simulink model "process_plant_model_4dof"  (R2020a)
settings: Solver=VariableStepAuto  StartTime=0.0  StopTime=10.0  RelTol=1e-3
values from neighbouring files (symbols this model uses):
  B_aug = [b11 b12 b13 b14 b15 b16 ... (first row only)    [constants.m]
  B_psinv_aug = B_aug'/(B_aug*B_aug')    [constants.m]
  coriolis_effect = 1    [run_simulation.m]    (also in run_simulation_STA_controller.m; run_simulation_dp_model.m)
  d_11 = 250    [constants.m]    (also in constants_dp_model.m; constants_model_coriolis.m; constants_process_model.m)
  d_22 = 200    [constants.m]    (also in constants_dp_model.m; constants_model_coriolis.m; constants_process_model.m)
  d_33 = 175    [constants.m]    (also in constants_dp_model.m; constants_model_coriolis.m; constants_process_model.m)
  d_66 = 15    [constants.m]    (also in constants_process_model.m)
  d_n11 = 350    [constants.m]
  d_n22 = 350    [constants.m]
  d_n33 = 400    [constants.m]
  d_n66 = 75    [constants.m]
  g_z = 9.81    [run_simulation_FL_controller.m]    (also in run_simulation_PID_controller.m = 0.91; run_simulation_SM_controller.m = 0.91; run_simulation_STA_controller.m = 0.91; run_simulation_dp_model.m = 0.91)
  m_11 = m_RB11+m_A11    (= 144)    [constants.m]    (also in constants_dp_model.m; constants_model_coriolis.m; constants_process_model.m)
  m_22 = m_RB22+m_A22    (= 162)    [constants.m]    (also in constants_dp_model.m; constants_model_coriolis.m; constants_process_model.m)
  m_A11 = 54    [constants.m]    (also in constants_dp_model.m; constants_model_coriolis.m; constants_process_model.m)
  m_A22 = 72    [constants.m]    (also in constants_dp_model.m; constants_model_coriolis.m; constants_process_model.m)
  m_A33 = 360    [constants.m]    (also in constants_dp_model.m; constants_model_coriolis.m; constants_process_model.m)
  m_A66 = 5.2    [constants.m]    (also in constants_process_model.m)
  m_RB11 = 90    [constants.m]    (also in constants_dp_model.m; constants_model_coriolis.m; constants_process_model.m)
  m_RB22 = 90    [constants.m]    (also in constants_dp_model.m; constants_model_coriolis.m; constants_process_model.m)
  m_RB33 = 90    [constants.m]    (also in constants_dp_model.m; constants_model_coriolis.m; constants_process_model.m)
  m_RB66 = 13    [constants.m]    (also in constants_process_model.m)
  nonlinear_damping = 1    [run_simulation.m]    (also in run_simulation_STA_controller.m; run_simulation_dp_model.m)
  psi0 = deg2rad(psi0)    [constants.m]    (also in constants_dp_model.m; constants_model_coriolis.m; constants_process_model.m)
  r0 = 0    [constants.m]    (also in constants_dp_model.m; constants_model_coriolis.m; constants_process_model.m)
  u0 = 0    [constants.m]    (also in constants_dp_model.m; constants_model_coriolis.m; constants_process_model.m)
  v0 = 0    [constants.m]    (also in constants_dp_model.m; constants_model_coriolis.m; constants_process_model.m)
  w0 = 0    [constants.m]    (also in constants_dp_model.m; constants_model_coriolis.m; constants_process_model.m)
  x0 = -2*50    (= -100)    [constants.m]    (also in constants_dp_model.m = 0; constants_model_coriolis.m = 0; constants_process_model.m = 0)
  y0 = 0    [constants.m]    (also in constants_dp_model.m; constants_model_coriolis.m; constants_process_model.m)
  z0 = 0    [constants.m]    (also in constants_dp_model.m; constants_model_coriolis.m; constants_process_model.m)
settings Model: Creator=kenng  LastModifiedBy=kennyhn

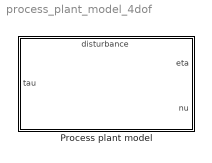
== system process_plant_model_4dof ==
  Process plant model : Subsystem
      settings: PortSchema="{\"entries\":[{\"content\":{\"sides\":[{\"content\":{\"connectorIds\":[\"In1\"]},\"type\":\"ConnectorPlacement.EquallySpacedRectSide\",\"uuid\":\"e717a587-3200-458e-ba24-dd41565550b9\"},{\"content\":{\"connectorIds\":[\"Out1\",\"Out2\"],\"side\":\"RIGHT\"},\"type\":\"ConnectorPlacement.EquallySpacedRectSide\",\"uuid\":\"302c9cc9-c34e-45c2-bf93-40982187bd66\"},{\"content\":{\"connectorIds\":[\"In2\"],\"side\":\"TOP\"},\"type\":\"ConnectorPlacement.EquallySpacedRectSide\",\"uuid\":\"4b1c13ad-6fa1-447d-8a08-ad292496a8ea\"}]},\"type\":\"ConnectorPlacement.EquallySpacedConnector\",\"uuid\":\"78ff5622-69b9-4402-ac71-5e2cc2861626\"}],\"packageUris\":[\"http://schema.mathworks.com/mf0/Connector/19700101\"],\"version\":\"1.0\"}"

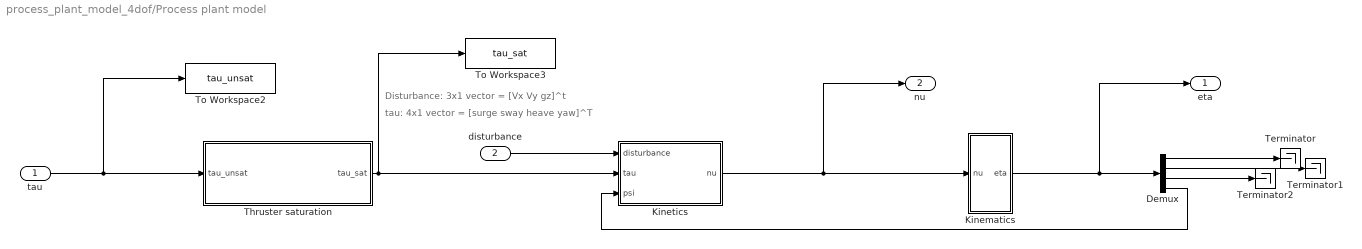
== system process_plant_model_4dof/Process plant model ==
  note: tau: 4x1 vector = [surge sway heave yaw]^T
  note: Disturbance: 3x1 vector = [Vx Vy gz]^t
  tau : Inport
  disturbance : Inport  Port=2
  Demux : Demux
  Kinematics : Subsystem
  Kinetics : Subsystem
  Terminator : Terminator
  Terminator1 : Terminator
  Terminator2 : Terminator
  Thruster saturation : Subsystem
  To Workspace2 : ToWorkspace  VariableName=tau_unsat  SaveFormat=Structure With Time  SampleTime=-1
  To Workspace3 : ToWorkspace  VariableName=tau_sat  SaveFormat=Structure With Time  SampleTime=-1
  eta : Outport
  nu : Outport  Port=2
  wires:
  Kinetics/1(nu) -> nu/1, Kinematics/1(nu)
  Demux/4 -> Kinetics/3(psi)
  Demux/2 -> Terminator1/1
  Kinematics/1(eta) -> eta/1, Demux/1
  Demux/1 -> Terminator/1
  Demux/3 -> Terminator2/1
  disturbance/1 -> Kinetics/1(disturbance)
  Thruster saturation/1(tau_sat) -> Kinetics/2(tau), To Workspace3/1
  tau/1 -> Thruster saturation/1(tau_unsat), To Workspace2/1

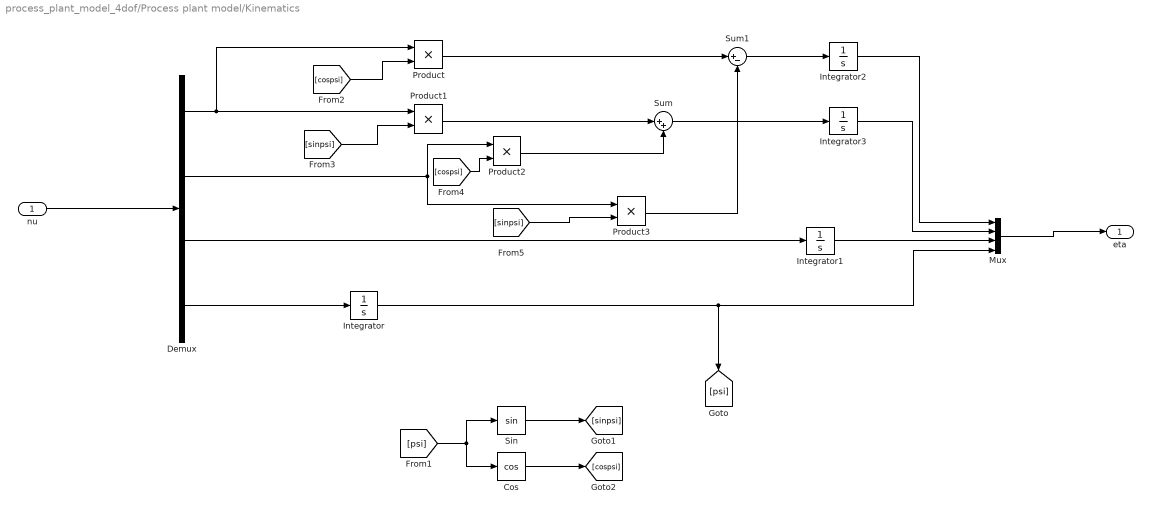
== system process_plant_model_4dof/Process plant model/Kinematics ==
  nu : Inport
  Cos : Trigonometry  Operator=cos
  Demux : Demux
  Integrator : Integrator  InitialCondition=psi0
  Integrator1 : Integrator  InitialCondition=z0
  Integrator2 : Integrator  InitialCondition=x0
  Integrator3 : Integrator  InitialCondition=y0
  Mux : Mux
  Product{,1..3} (4 alike) : Product
  Sin : Trigonometry
  Sum : Sum  Inputs=|++
  Sum1 : Sum  Inputs=|+-
  eta : Outport
  wires:
  Sin/1 -> [sinpsi]
  Demux/3 -> Integrator1/1
  Demux/1 -> Product1/1, Product/1
  Demux/2 -> Product3/1, Product2/1
  [sinpsi] -> Product3/2
  [psi] -> Sin/1, Cos/1
  [cospsi] -> Product2/2
  Cos/1 -> [cospsi]
  Product1/1 -> Sum/1
  Integrator/1 -> Mux/4, [psi]
  [sinpsi] -> Product1/2
  Product/1 -> Sum1/1
  Sum1/1 -> Integrator2/1
  Demux/4 -> Integrator/1
  Sum/1 -> Integrator3/1
  [cospsi] -> Product/2
  nu/1 -> Demux/1
  Product2/1 -> Sum/2
  Product3/1 -> Sum1/2
  Integrator3/1 -> Mux/2
  Integrator1/1 -> Mux/3
  Integrator2/1 -> Mux/1
  Mux/1 -> eta/1

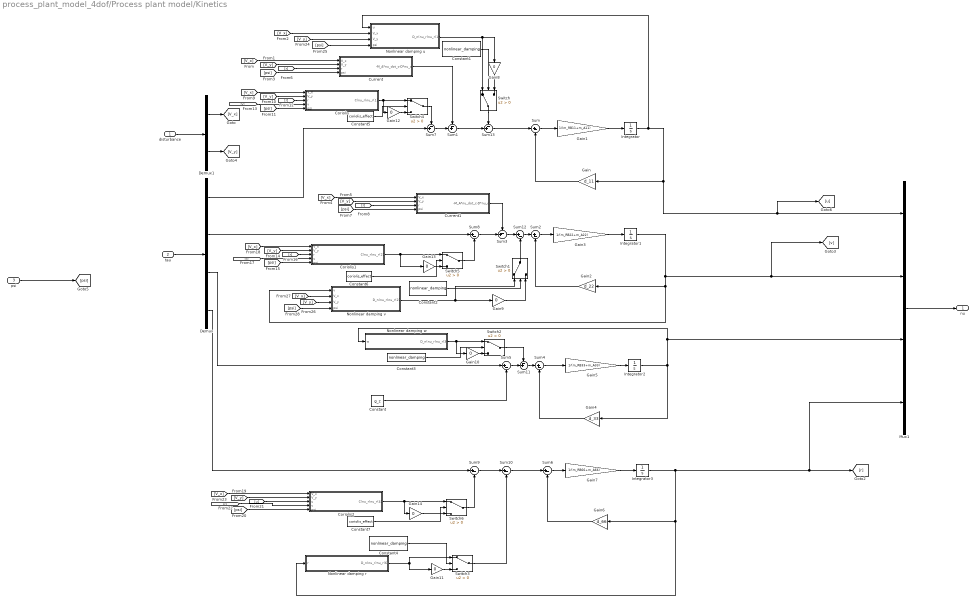
== system process_plant_model_4dof/Process plant model/Kinetics ==
  disturbance : Inport
  tau : Inport  Port=2
  psi : Inport  Port=3
  Constant : Constant  Value=g_z
  Constant{1..4} (4 alike) : Constant  Value=nonlinear_damping
  Constant5 : Constant  Value=coriolis_effect
  Constant6 : Constant  Value=coriolis_effect
  Constant7 : Constant  Value=coriolis_effect
  Coriolis : Subsystem
  Coriolis1 : Subsystem
  Coriolis2 : Subsystem
  Current : Subsystem
  Current1 : Subsystem
  Demux : Demux
  Demux1 : Demux  Outputs=2
  Gain : Gain  Gain=d_11
  Gain1 : Gain  Gain=1/(m_RB11+m_A11)
  Gain{8..14} (7 alike) : Gain  Gain=0
  Gain2 : Gain  Gain=d_22
  Gain3 : Gain  Gain=1/(m_RB22+m_A22)
  Gain4 : Gain  Gain=d_33
  Gain5 : Gain  Gain=1/(m_RB33+m_A33)
  Gain6 : Gain  Gain=d_66
  Gain7 : Gain  Gain=1/(m_RB66+m_A66)
  Integrator : Integrator  InitialCondition=u0
  Integrator1 : Integrator  InitialCondition=v0
  Integrator2 : Integrator  InitialCondition=w0
  Integrator3 : Integrator  InitialCondition=r0
  Mux1 : Mux
  Nonlinear damping r : Subsystem
  Nonlinear damping u : Subsystem
  Nonlinear damping v : Subsystem
  Nonlinear damping w : Subsystem
  Sum{,2,4..6,8..10,12} (9 alike) : Sum  Inputs=|+-
  Sum{1,3,7,11,13} (5 alike) : Sum  Inputs=-+|
  Switch{,1..6} (7 alike) : Switch  Criteria=u2 > Threshold
  nu : Outport
  wires:
  Demux1/1 -> [V_x]
  Gain1/1 -> Integrator/1
  Sum/1 -> Gain1/1
  tau/1 -> Demux/1
  Integrator1/1 -> Nonlinear damping v/1(v), Gain2/1, [v], Mux1/2
  Gain3/1 -> Integrator1/1
  Mux1/1 -> nu/1
  Integrator/1 -> Nonlinear damping u/1(u), [u], Mux1/1, Gain/1
  Integrator2/1 -> Gain4/1, Nonlinear damping w/1(w), Mux1/3
  Gain5/1 -> Integrator2/1
  Sum4/1 -> Gain5/1
  Gain2/1 -> Sum2/2
  Sum2/1 -> Gain3/1
  Gain/1 -> Sum/2
  Gain4/1 -> Sum4/2
  Gain6/1 -> Sum6/2
  Demux1/2 -> [V_y]
  [r] -> Current/3(r)
  Integrator3/1 -> [r], Mux1/4, Nonlinear damping r/1(r), Gain6/1
  disturbance/1 -> Demux1/1
  Sum6/1 -> Gain7/1
  Gain7/1 -> Integrator3/1
  psi/1 -> [psi]
  Current/1(-M_A*nu_dot_c-D*nu_c) -> Sum1/1
  [V_y] -> Current/2(V_y)
  [V_x] -> Current/1(V_x)
  [psi] -> Current/4(psi)
  [r] -> Current1/3(r)
  [psi] -> Current1/4(psi)
  [V_x] -> Current1/1(V_x)
  [V_y] -> Current1/2(V_y)
  Current1/1(-M_A*nu_dot_c-D*nu_c) -> Sum3/1
  Constant/1 -> Sum5/2
  Demux/3 -> Sum5/1
  Demux/1 -> Sum7/2
  Sum7/1 -> Sum1/2
  [V_x] -> Coriolis/1(V_x)
  [psi] -> Coriolis/5(psi)
  [r] -> Coriolis/3(r)
  [V_y] -> Coriolis/2(V_y)
  [v] -> Coriolis/4(v)
  [u] -> Coriolis1/4(u)
  [V_y] -> Coriolis1/2(V_y)
  [psi] -> Coriolis1/5(psi)
  [V_x] -> Coriolis1/1(V_x)
  [r] -> Coriolis1/3(r)
  Sum8/1 -> Sum3/2
  Demux/2 -> Sum8/1
  [v] -> Coriolis2/4(v)
  [V_y] -> Coriolis2/2(V_y)
  [psi] -> Coriolis2/5(psi)
  [V_x] -> Coriolis2/1(V_x)
  [u] -> Coriolis2/3(u)
  Demux/4 -> Sum9/1
  Sum10/1 -> Sum6/1
  Sum5/1 -> Sum11/2
  Sum11/1 -> Sum4/1
  Nonlinear damping w/1(D_n(nu_r)nu_r(3)) -> Gain10/1, Switch2/1
  Sum12/1 -> Sum2/1
  Sum1/1 -> Sum13/2
  Sum13/1 -> Sum/1
  Nonlinear damping u/1(D_n(nu_r)nu_r(1)) -> Switch/1, Gain8/1
  [V_x] -> Nonlinear damping u/2(V_x)
  [V_y] -> Nonlinear damping u/3(V_y)
  [psi] -> Nonlinear damping u/4(psi)
  Sum3/1 -> Sum12/1
  Nonlinear damping v/1(D_n(nu_r)nu_r(2)) -> Gain9/1, Switch1/1
  [V_x] -> Nonlinear damping v/2(V_x)
  [V_y] -> Nonlinear damping v/3(V_y)
  [psi] -> Nonlinear damping v/4(psi)
  Sum9/1 -> Sum10/1
  Switch/1 -> Sum13/1
  Switch1/1 -> Sum12/2
  Switch2/1 -> Sum11/1
  Switch3/1 -> Sum10/2
  Constant1/1 -> Switch/2
  Gain8/1 -> Switch/3
  Gain9/1 -> Switch1/3
  Constant2/1 -> Switch1/2
  Gain10/1 -> Switch2/3
  Constant3/1 -> Switch2/2
  Gain11/1 -> Switch3/3
  Constant4/1 -> Switch3/2
  Nonlinear damping r/1(D_n(nu_r)nu_r(6)) -> Switch3/1, Gain11/1
  Switch4/1 -> Sum7/1
  Coriolis/1(C(nu_r)nu_r(1)) -> Switch4/1, Gain12/1
  Constant5/1 -> Switch4/2
  Gain12/1 -> Switch4/3
  Switch5/1 -> Sum8/2
  Gain13/1 -> Switch5/3
  Constant6/1 -> Switch5/2
  Coriolis1/1(C(nu_r)nu_r(2)) -> Switch5/1, Gain13/1
  Coriolis2/1(C(nu_r)nu_r(4)) -> Switch6/1, Gain14/1
  Switch6/1 -> Sum9/2
  Gain14/1 -> Switch6/3
  Constant7/1 -> Switch6/2

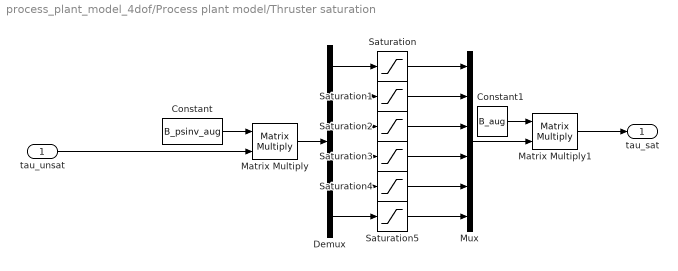
== system process_plant_model_4dof/Process plant model/Thruster saturation ==
  tau_unsat : Inport
  Constant : Constant  Value=B_psinv_aug
  Constant1 : Constant  Value=B_aug
  Demux : Demux  Outputs=6
  Matrix Multiply : Product  Multiplication=Matrix(*)
  Matrix Multiply1 : Product  Multiplication=Matrix(*)
  Mux : Mux  Inputs=6
  Saturation{,1..5} (6 alike) : Saturate  UpperLimit=120  LowerLimit=-120
  tau_sat : Outport
  wires:
  tau_unsat/1 -> Matrix Multiply/2
  Constant/1 -> Matrix Multiply/1
  Matrix Multiply/1 -> Demux/1
  Demux/2 -> Saturation1/1
  Demux/1 -> Saturation/1
  Demux/3 -> Saturation2/1
  Demux/4 -> Saturation3/1
  Demux/5 -> Saturation4/1
  Demux/6 -> Saturation5/1
  Saturation/1 -> Mux/1
  Saturation1/1 -> Mux/2
  Saturation2/1 -> Mux/3
  Saturation3/1 -> Mux/4
  Saturation4/1 -> Mux/5
  Saturation5/1 -> Mux/6
  Mux/1 -> Matrix Multiply1/2
  Constant1/1 -> Matrix Multiply1/1
  Matrix Multiply1/1 -> tau_sat/1

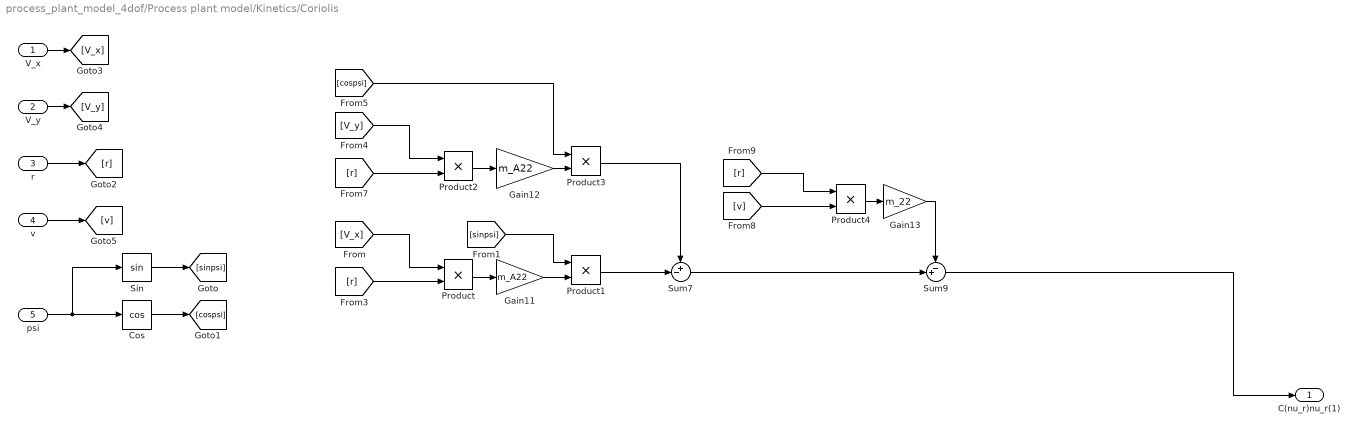
== system process_plant_model_4dof/Process plant model/Kinetics/Coriolis ==
  V_x : Inport
  V_y : Inport  Port=2
  r : Inport  Port=3
  v : Inport  Port=4
  psi : Inport  Port=5
  Cos : Trigonometry  Operator=cos
  Gain11 : Gain  Gain=m_A22
  Gain12 : Gain  Gain=m_A22
  Gain13 : Gain  Gain=m_22
  Product{,1..4} (5 alike) : Product
  Sin : Trigonometry
  Sum7 : Sum  Inputs=+-|
  Sum9 : Sum  Inputs=-+|
  C(nu_r)nu_r(1) : Outport
  wires:
  Gain11/1 -> Product1/2
  Product2/1 -> Gain12/1
  [cospsi] -> Product3/1
  [r] -> Product2/2
  [v] -> Product4/2
  Product4/1 -> Gain13/1
  [V_x] -> Product/1
  Product3/1 -> Sum7/1
  Gain12/1 -> Product3/2
  Product/1 -> Gain11/1
  [V_y] -> Product2/1
  [r] -> Product/2
  Product1/1 -> Sum7/2
  [sinpsi] -> Product1/1
  Sum7/1 -> Sum9/2
  [r] -> Product4/1
  Sum9/1 -> C(nu_r)nu_r(1)/1
  psi/1 -> Sin/1, Cos/1
  Sin/1 -> [sinpsi]
  Cos/1 -> [cospsi]
  r/1 -> [r]
  V_x/1 -> [V_x]
  V_y/1 -> [V_y]
  v/1 -> [v]
  Gain13/1 -> Sum9/1

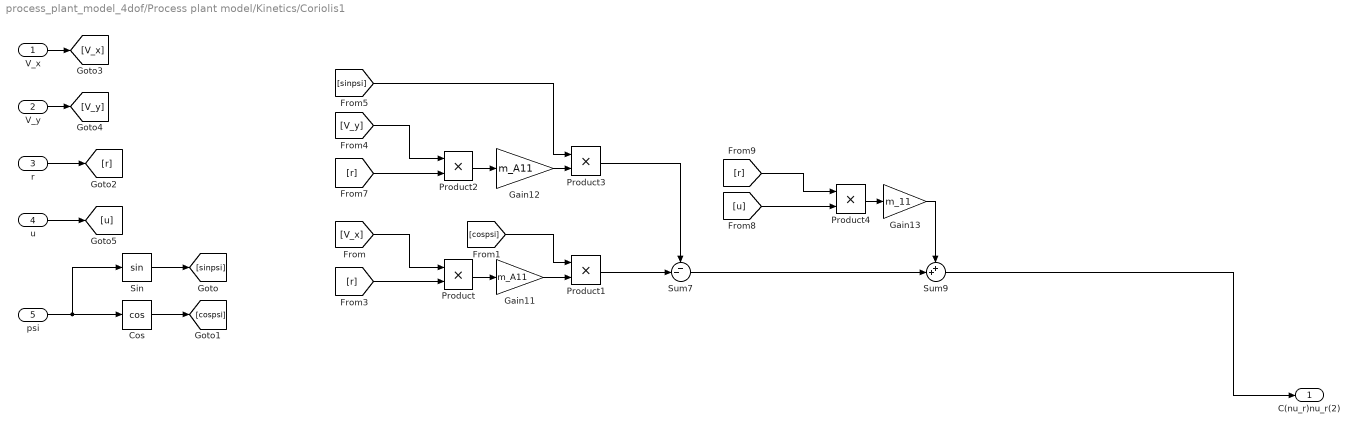
== system process_plant_model_4dof/Process plant model/Kinetics/Coriolis1 ==
  V_x : Inport
  V_y : Inport  Port=2
  r : Inport  Port=3
  u : Inport  Port=4
  psi : Inport  Port=5
  Cos : Trigonometry  Operator=cos
  Gain11 : Gain  Gain=m_A11
  Gain12 : Gain  Gain=m_A11
  Gain13 : Gain  Gain=m_11
  Product{,1..4} (5 alike) : Product
  Sin : Trigonometry
  Sum7 : Sum  Inputs=--|
  Sum9 : Sum  Inputs=++|
  C(nu_r)nu_r(2) : Outport
  wires:
  Gain11/1 -> Product1/2
  Product2/1 -> Gain12/1
  [sinpsi] -> Product3/1
  [r] -> Product2/2
  [u] -> Product4/2
  Product4/1 -> Gain13/1
  [V_x] -> Product/1
  Product3/1 -> Sum7/1
  Gain12/1 -> Product3/2
  Product/1 -> Gain11/1
  [V_y] -> Product2/1
  [r] -> Product/2
  Product1/1 -> Sum7/2
  [cospsi] -> Product1/1
  Sum7/1 -> Sum9/2
  [r] -> Product4/1
  Sum9/1 -> C(nu_r)nu_r(2)/1
  psi/1 -> Sin/1, Cos/1
  Sin/1 -> [sinpsi]
  Cos/1 -> [cospsi]
  r/1 -> [r]
  V_x/1 -> [V_x]
  V_y/1 -> [V_y]
  u/1 -> [u]
  Gain13/1 -> Sum9/1

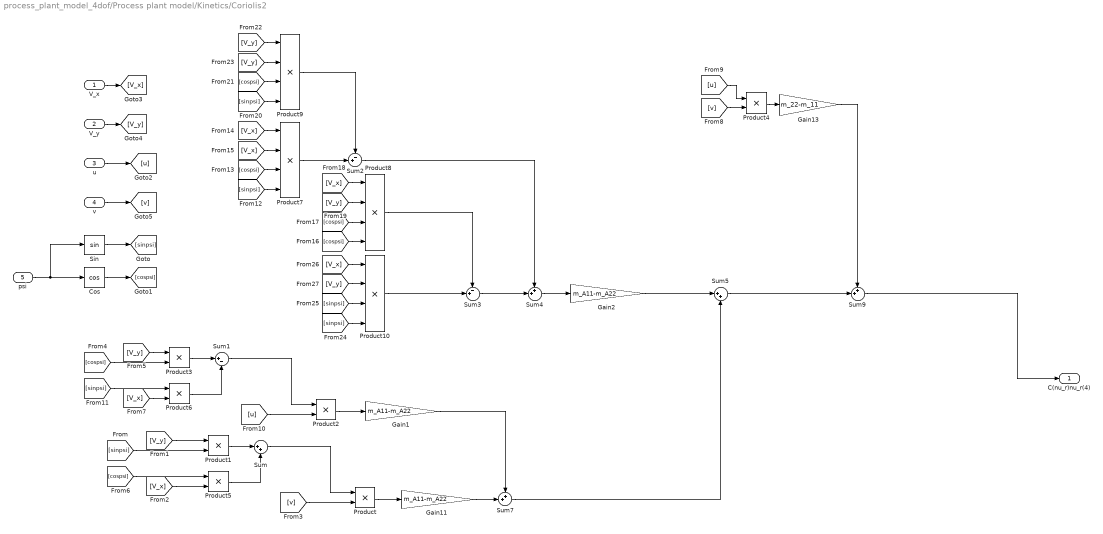
== system process_plant_model_4dof/Process plant model/Kinetics/Coriolis2 ==
  V_x : Inport
  V_y : Inport  Port=2
  u : Inport  Port=3
  v : Inport  Port=4
  psi : Inport  Port=5
  Cos : Trigonometry  Operator=cos
  Gain1 : Gain  Gain=m_A11-m_A22
  Gain11 : Gain  Gain=m_A11-m_A22
  Gain13 : Gain  Gain=m_22-m_11
  Gain2 : Gain  Gain=m_A11-m_A22
  Product{,1..6} (7 alike) : Product
  Product{7..10} (4 alike) : Product  Inputs=4
  Sin : Trigonometry
  Sum : Sum  Inputs=|++
  Sum1 : Sum  Inputs=|+-
  Sum2 : Sum  Inputs=-+|
  Sum3 : Sum  Inputs=-+|
  Sum4 : Sum  Inputs=++|
  Sum5 : Sum  Inputs=|++
  Sum7 : Sum  Inputs=++|
  Sum9 : Sum  Inputs=++|
  C(nu_r)nu_r(4) : Outport
  wires:
  [v] -> Product4/2
  Product4/1 -> Gain13/1
  Product/1 -> Gain11/1
  [v] -> Product/2
  Gain11/1 -> Sum7/2
  [u] -> Product4/1
  Sum9/1 -> C(nu_r)nu_r(4)/1
  psi/1 -> Sin/1, Cos/1
  Sin/1 -> [sinpsi]
  Cos/1 -> [cospsi]
  u/1 -> [u]
  V_x/1 -> [V_x]
  V_y/1 -> [V_y]
  v/1 -> [v]
  Gain13/1 -> Sum9/1
  [V_y] -> Product1/1
  [V_x] -> Product5/2
  Product1/1 -> Sum/1
  Product5/1 -> Sum/2
  Sum/1 -> Product/1
  [sinpsi] -> Product1/2
  [cospsi] -> Product5/1
  Product2/1 -> Gain1/1
  [u] -> Product2/2
  [V_x] -> Product6/2
  Sum1/1 -> Product2/1
  [cospsi] -> Product3/2
  [V_y] -> Product3/1
  [sinpsi] -> Product6/1
  Product3/1 -> Sum1/1
  Product6/1 -> Sum1/2
  Gain1/1 -> Sum7/1
  [sinpsi] -> Product7/4
  [cospsi] -> Product7/3
  [V_x] -> Product7/1
  [V_x] -> Product7/2
  [sinpsi] -> Product9/4
  [V_y] -> Product9/1
  [cospsi] -> Product9/3
  [V_y] -> Product9/2
  Product7/1 -> Sum2/2
  Product9/1 -> Sum2/1
  [V_y] -> Product8/2
  [cospsi] -> Product8/3
  [V_x] -> Product8/1
  Product8/1 -> Sum3/1
  [cospsi] -> Product8/4
  [V_y] -> Product10/2
  [sinpsi] -> Product10/3
  [V_x] -> Product10/1
  [sinpsi] -> Product10/4
  Product10/1 -> Sum3/2
  Sum3/1 -> Sum4/2
  Sum2/1 -> Sum4/1
  Sum4/1 -> Gain2/1
  Sum7/1 -> Sum5/2
  Sum5/1 -> Sum9/2
  Gain2/1 -> Sum5/1

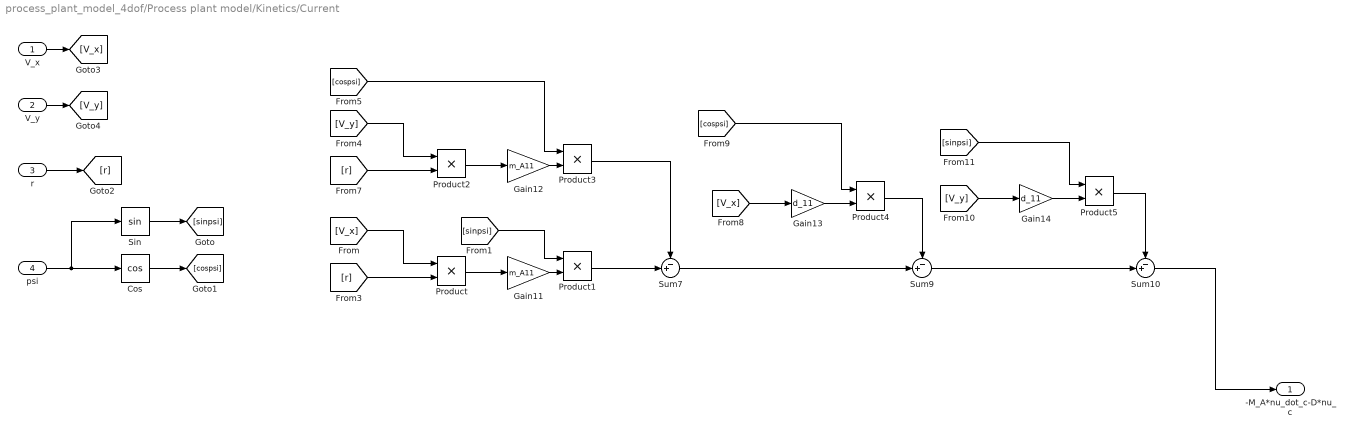
== system process_plant_model_4dof/Process plant model/Kinetics/Current ==
  V_x : Inport
  V_y : Inport  Port=2
  r : Inport  Port=3
  psi : Inport  Port=4
  Cos : Trigonometry  Operator=cos
  Gain11 : Gain  Gain=m_A11
  Gain12 : Gain  Gain=m_A11
  Gain13 : Gain  Gain=d_11
  Gain14 : Gain  Gain=d_11
  Product{,1..5} (6 alike) : Product
  Sin : Trigonometry
  Sum10 : Sum  Inputs=-+|
  Sum7 : Sum  Inputs=-+|
  Sum9 : Sum  Inputs=-+|
  -M_A*nu_dot_c-D*nu_c : Outport
  wires:
  Gain11/1 -> Product1/2
  Product2/1 -> Gain12/1
  [cospsi] -> Product3/1
  [r] -> Product2/2
  Gain13/1 -> Product4/2
  Product4/1 -> Sum9/1
  [V_x] -> Product/1
  Product3/1 -> Sum7/1
  Gain12/1 -> Product3/2
  Product/1 -> Gain11/1
  [V_y] -> Product2/1
  [r] -> Product/2
  Product1/1 -> Sum7/2
  [sinpsi] -> Product1/1
  Gain14/1 -> Product5/2
  [sinpsi] -> Product5/1
  Sum7/1 -> Sum9/2
  [cospsi] -> Product4/1
  [V_y] -> Gain14/1
  [V_x] -> Gain13/1
  Product5/1 -> Sum10/1
  Sum9/1 -> Sum10/2
  Sum10/1 -> -M_A*nu_dot_c-D*nu_c/1
  psi/1 -> Sin/1, Cos/1
  Sin/1 -> [sinpsi]
  Cos/1 -> [cospsi]
  r/1 -> [r]
  V_x/1 -> [V_x]
  V_y/1 -> [V_y]

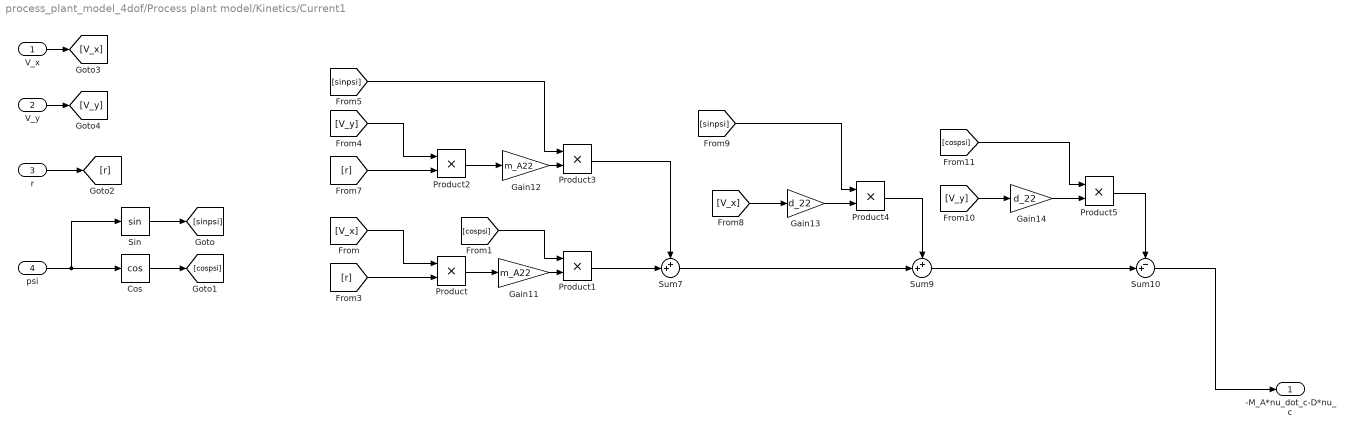
== system process_plant_model_4dof/Process plant model/Kinetics/Current1 ==
  V_x : Inport
  V_y : Inport  Port=2
  r : Inport  Port=3
  psi : Inport  Port=4
  Cos : Trigonometry  Operator=cos
  Gain11 : Gain  Gain=m_A22
  Gain12 : Gain  Gain=m_A22
  Gain13 : Gain  Gain=d_22
  Gain14 : Gain  Gain=d_22
  Product{,1..5} (6 alike) : Product
  Sin : Trigonometry
  Sum10 : Sum  Inputs=-+|
  Sum7 : Sum  Inputs=++|
  Sum9 : Sum  Inputs=++|
  -M_A*nu_dot_c-D*nu_c : Outport
  wires:
  Gain11/1 -> Product1/2
  Product2/1 -> Gain12/1
  [sinpsi] -> Product3/1
  [r] -> Product2/2
  Gain13/1 -> Product4/2
  Product4/1 -> Sum9/1
  [V_x] -> Product/1
  Product3/1 -> Sum7/1
  Gain12/1 -> Product3/2
  Product/1 -> Gain11/1
  [V_y] -> Product2/1
  [r] -> Product/2
  Product1/1 -> Sum7/2
  [cospsi] -> Product1/1
  Gain14/1 -> Product5/2
  [cospsi] -> Product5/1
  Sum7/1 -> Sum9/2
  [sinpsi] -> Product4/1
  [V_y] -> Gain14/1
  [V_x] -> Gain13/1
  Product5/1 -> Sum10/1
  Sum9/1 -> Sum10/2
  Sum10/1 -> -M_A*nu_dot_c-D*nu_c/1
  psi/1 -> Sin/1, Cos/1
  Sin/1 -> [sinpsi]
  Cos/1 -> [cospsi]
  r/1 -> [r]
  V_x/1 -> [V_x]
  V_y/1 -> [V_y]

== system process_plant_model_4dof/Process plant model/Kinetics/Nonlinear damping r ==
  r : Inport
  Abs : Abs
  Gain : Gain  Gain=d_n66
  Product : Product
  D_n(nu_r)nu_r(6) : Outport
  wires:
  Abs/1 -> Gain/1
  Product/1 -> D_n(nu_r)nu_r(6)/1
  Gain/1 -> Product/1
  r/1 -> Abs/1, Product/2

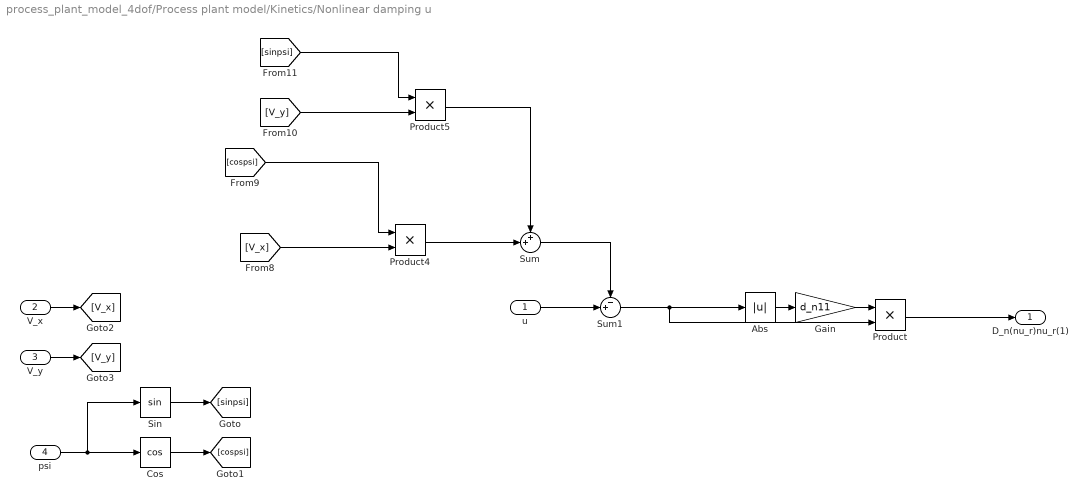
== system process_plant_model_4dof/Process plant model/Kinetics/Nonlinear damping u ==
  u : Inport
  V_x : Inport  Port=2
  V_y : Inport  Port=3
  psi : Inport  Port=4
  Abs : Abs
  Cos : Trigonometry  Operator=cos
  Gain : Gain  Gain=d_n11
  Product : Product
  Product4 : Product
  Product5 : Product
  Sin : Trigonometry
  Sum : Sum  Inputs=++|
  Sum1 : Sum  Inputs=-+|
  D_n(nu_r)nu_r(1) : Outport
  wires:
  Gain/1 -> Product/1
  Product/1 -> D_n(nu_r)nu_r(1)/1
  Abs/1 -> Gain/1
  psi/1 -> Sin/1, Cos/1
  Sin/1 -> [sinpsi]
  Cos/1 -> [cospsi]
  [V_y] -> Product5/2
  [sinpsi] -> Product5/1
  Product4/1 -> Sum/2
  [V_x] -> Product4/2
  [cospsi] -> Product4/1
  Product5/1 -> Sum/1
  V_x/1 -> [V_x]
  V_y/1 -> [V_y]
  u/1 -> Sum1/2
  Sum1/1 -> Product/2, Abs/1
  Sum/1 -> Sum1/1

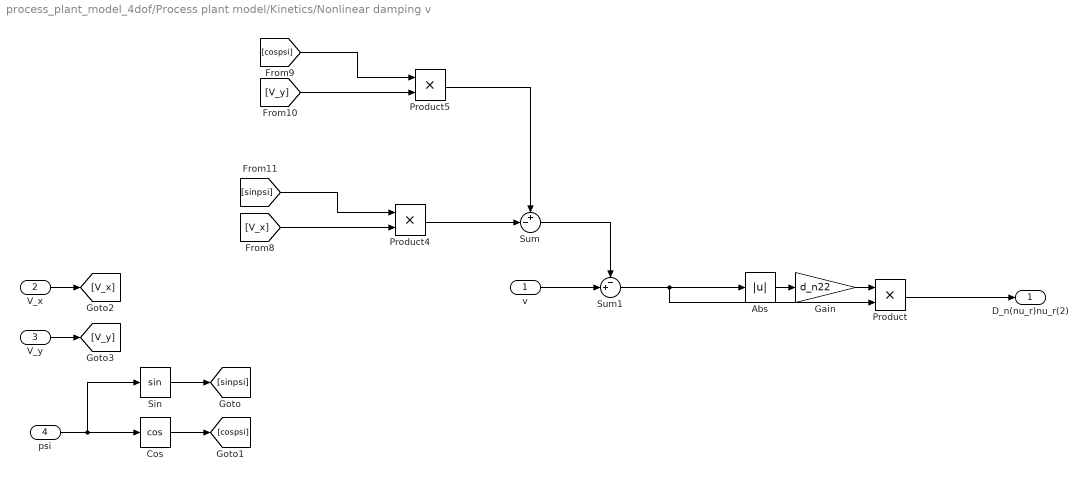
== system process_plant_model_4dof/Process plant model/Kinetics/Nonlinear damping v ==
  v : Inport
  V_x : Inport  Port=2
  V_y : Inport  Port=3
  psi : Inport  Port=4
  Abs : Abs
  Cos : Trigonometry  Operator=cos
  Gain : Gain  Gain=d_n22
  Product : Product
  Product4 : Product
  Product5 : Product
  Sin : Trigonometry
  Sum : Sum  Inputs=+-|
  Sum1 : Sum  Inputs=-+|
  D_n(nu_r)nu_r(2) : Outport
  wires:
  Gain/1 -> Product/1
  Product/1 -> D_n(nu_r)nu_r(2)/1
  Abs/1 -> Gain/1
  psi/1 -> Sin/1, Cos/1
  Sin/1 -> [sinpsi]
  Cos/1 -> [cospsi]
  [V_y] -> Product5/2
  Product4/1 -> Sum/2
  [V_x] -> Product4/2
  Product5/1 -> Sum/1
  V_x/1 -> [V_x]
  V_y/1 -> [V_y]
  v/1 -> Sum1/2
  Sum1/1 -> Product/2, Abs/1
  Sum/1 -> Sum1/1
  [sinpsi] -> Product4/1
  [cospsi] -> Product5/1

== system process_plant_model_4dof/Process plant model/Kinetics/Nonlinear damping w ==
  w : Inport
  Abs : Abs
  Gain : Gain  Gain=d_n33
  Product : Product
  D_n(nu_r)nu_r(3) : Outport
  wires:
  Abs/1 -> Gain/1
  Product/1 -> D_n(nu_r)nu_r(3)/1
  Gain/1 -> Product/1
  w/1 -> Abs/1, Product/2
